simulink model "RobotX_ss_acousticsSingle_Dock_1023"  (R2014a)
settings: Solver=FixedStepDiscrete  StartTime=0.0  StopTime=inf  FixedStep=.25  RelTol=1e-3
undefined symbols (not defined in the file): Com1, Com2, Com3, Com4, DiscIntNeverNeededParam, standard
libraries: xpcseriallib x42, slrtlib x7, simulink x6, speedgoatlib x2, dspmtrx3 x1, speedgoatlib_IO102 x1
(part 4 of 4)

== matlab function RobotX_ss_acousticsSingle_Dock_1023/Sensors/1021 Comms/Message Selector/HRTSEA Message/MATLAB Function ==
  data: Time input; HRTLat input; HRTLong input; HRTTask input; HRTMode input; SEAValid input; asciiHRTSEA output; SEALat input; SEALong input; SEAColor input; SEADepth input
function asciiHRTSEA = asciiHRTSEAEncoder(Time,HRTLat,HRTLong,HRTTask,HRTMode,SEAValid,SEALat,SEALong,SEAColor,SEADepth)

% Initialize output message vector as the serial output block expects 128
% character message
asciiHRTSEA = uint8(zeros(1,128));

asciiComma = uint8(',');
asciiDeciPt = uint8('.');
asciiTeamID = uint8('FAUVU,');
asciiMsgEnd = uint8('*');
asciiMsgCRLF = [13 10];

% Convert UTC Time input (hhmmss) into ascii code
asciiTime = uint8(zeros(1,7));
asciiTime(7) = asciiComma;

for timeChar = 1:6
    asciiTime(timeChar) = floor(mod(Time,10^(7-timeChar))/...
        10^(6-timeChar)) + 48;
end

%%%%%%%%%%%%%%%%%%%%%%%%%%%%%%%%%%%%%%%%%%%%%%%%%%%%%%%%%%%%%%%%%%%%
% Heartbeat message
% Convert static strings to ascii code
asciiHRTMsgID = uint8('$RXHRT,');
if HRTLat >= 0
    asciiHRTNS = uint8('N,');
else
    HRTLat = -HRTLat;
    asciiHRTNS = uint8('S,');
end
if HRTLong >= 0
    asciiHRTEW = uint8('E,');
else
    HRTLong = -HRTLong;
    asciiHRTEW = uint8('W,');
end

% Convert latitude (dd.mmmmmm) into ascii code
asciiHRTLat = uint8(zeros(1,10));
asciiHRTLat(10) = asciiComma;
asciiHRTLat(3) = asciiDeciPt;

HRTlatInt = floor(HRTLat);
for latIntChar = 1:2
    asciiHRTLat(latIntChar) = floor(mod(HRTlatInt,10^(3-latIntChar))/...
        10^(2-latIntChar)) + 48;
end

HRTlatDeci = mod(HRTLat,HRTlatInt) * 10^6;
for latDeciChar = 1:6
    asciiHRTLat(latDeciChar+3) = floor(mod(HRTlatDeci,10^(7-latDeciChar))/...
        10^(6-latDeciChar)) + 48;
end

% Convert longitude (ddd.mmmmmm) into ascii code
asciiHRTLong = uint8(zeros(1,11));
asciiHRTLong(11) = asciiComma;
asciiHRTLong(4) = asciiDeciPt;

HRTlongInt = floor(HRTLong);
for longIntChar = 1:3
    asciiHRTLong(longIntChar) = floor(mod(HRTlongInt,10^(4-longIntChar))/...
        10^(3-longIntChar)) + 48;
end

HRTlongDeci = mod(HRTLong,HRTlongInt) * 10^6;
for longDeciChar = 1:6
    asciiHRTLong(longDeciChar+4) = floor(mod(HRTlongDeci,10^(7-longDeciChar))/...
        10^(6-longDeciChar)) + 48;
end

% Convert vehicle mode into ascii (1 = RC, 2 = Auto)

% Auto On 
if HRTMode == 3 
    HRTOpMode = 2;
    asciiHRTMode = [uint8(HRTOpMode+48) asciiComma];
else
    HRTOpMode = 1;
    asciiHRTMode = [uint8(HRTOpMode+48) asciiComma];
end

% Convert vehicle task into ascii
HRTTask = HRTTask - 1; % FSM: Init = 1, SSGate = 2, SEA = 3, Dock = 4, LIT = 5, Obst = 6
if HRTTask ~= 1 || 2 || 3 || 4 || 5
    HRTOpTask = 1;
    asciiHRTTask = [uint8(HRTOpTask+48) asciiMsgEnd];
else
    asciiHRTTask = [uint8(HRTTask+48) asciiMsgEnd];
end

% Concat individual ascii arrays into one array
asciiHRTPreChkSum = cat(2,asciiHRTMsgID,asciiTime,asciiHRTLat,asciiHRTNS,asciiHRTLong,asciiHRTEW,...
    asciiTeamID,asciiHRTMode,asciiHRTTask);

% Calculate the checksum of the message from the '$' to the '*' and convert
% to hex
HRTchkSum = uint8(0);

for chksumChar = 1:(length(asciiHRTPreChkSum)-2)
    HRTchkSum = bitxor(HRTchkSum,asciiHRTPreChkSum(chksumChar+1));
end

% Convert the checksum to ascii
HRTchkSum = dec2hex(HRTchkSum);
asciiHRTChkSum = uint8(zeros(1,length(HRTchkSum))+32);
for i = 1:length(HRTchkSum)
    asciiHRTChkSum(i) = uint8(HRTchkSum(i));
end

% Concat the checksum and the '/r/n' to the end of the message
asciiHRTPostChkSum = cat(2,asciiHRTPreChkSum,asciiHRTChkSum,asciiMsgCRLF);

%%%%%%%%%%%%%%%%%%%%%%%%%%%%%%%%%%%%%%%%%%%%%%%%%%%%%%%%%%%%%%%%%%%%%

% Underwater search message
asciiSEAMsgID = uint8('$RXSEA,');
if SEAValid == 1
    if SEALat >= 0
        asciiSEANS = uint8('N,');
    else
        SEALat = -SEALat;
        asciiSEANS = uint8('S,');
    end
    if SEALong >= 0
        asciiSEAEW = uint8('E,');
    else
        SEALong = -SEALong;
        asciiSEAEW = uint8('W,');
    end
else
    asciiSEANS = [32 asciiComma];
    asciiSEAEW = [32 asciiComma];
end

% Convert buoy color to ascii code (1 = R, 2 = G, 3 = B, 4 = W, 5 = K)
asciiSEAColor = [uint8(32) asciiComma]; % Initialize as whitespace in case no buoy is found

if SEAColor == 1
    asciiSEAColor(1) = uint8('R');
elseif SEAColor == 2
    asciiSEAColor(1) = uint8('G');
elseif SEAColor == 3
    asciiSEAColor(1) = uint8('B');
elseif SEAColor == 4
    asciiSEAColor(1) = uint8('W');
elseif SEAColor == 5
    asciiSEAColor(1) = uint8('K');
end

% Convert latitude (dd.mmmmmm) into ascii code
asciiSEALat = uint8(zeros(1,10)+32); % Initialize as whitespace in case no buoy is found
asciiSEALat(10) = asciiComma;

% Only output values if valid bit is high
if SEAValid == 1
    asciiSEALat(3) = asciiDeciPt;
    SEAlatInt = floor(SEALat);
    for latIntChar = 1:2
        asciiSEALat(latIntChar) = floor(mod(SEAlatInt,10^(3-latIntChar))/...
            10^(2-latIntChar)) + 48;
    end
    
    SEAlatDeci = mod(SEALat,SEAlatInt) * 10^6;
    for latDeciChar = 1:6
        asciiSEALat(latDeciChar+3) = floor(mod(SEAlatDeci,10^(7-latDeciChar))/...
            10^(6-latDeciChar)) + 48;
    end
end

% Convert longitude (ddd.mmmmmm) into ascii code
asciiSEALong = uint8(zeros(1,11)+32); % Initialize as whitespace in case no buoy is found
asciiSEALong(11) = asciiComma;

% Only output values if valid bit is high
if SEAValid == 1
    asciiSEALong(4) = asciiDeciPt;
    SEAlongInt = floor(SEALong);
    for longIntChar = 1:3
        asciiSEALong(longIntChar) = floor(mod(SEAlongInt,10^(4-longIntChar))/...
            10^(3-longIntChar)) + 48;
    end
    
    SEAlongDeci = mod(SEALong,SEAlongInt) * 10^6;
    for longDeciChar = 1:6
        asciiSEALong(longDeciChar+4) = floor(mod(SEAlongDeci,10^(7-longDeciChar))/...
            10^(6-longDeciChar)) + 48;
    end
end

% Convert depth (m) (##.##) into ascii
asciiSEADepth = uint8(zeros(1,6)+32); % Initialize as whitespace in case no buoy is found
asciiSEADepth(6) = asciiMsgEnd;

% Only output values if valid bit is high
if SEAValid == 1
    asciiSEADepth(3) = asciiDeciPt;
    SEAdepthInt = floor(SEADepth);
    for depthIntChar = 1:2
        asciiSEADepth(depthIntChar) = floor(mod(SEAdepthInt,10^(3-depthIntChar))/...
            10^(2-depthIntChar)) + 48;
    end
    
    SEAdepthDeci = mod(SEADepth,SEAdepthInt) * 10^2;
    for depthDeciChar = 1:2
        asciiSEADepth(depthDeciChar+3) = floor(mod(SEAdepthDeci,10^(3-depthDeciChar))/...
            10^(2-depthDeciChar)) + 48;
    end
end

% Concat individual ascii arrays into one array
asciiSEAPreChkSum = cat(2,asciiSEAMsgID,asciiTime,asciiTeamID,asciiSEAColor,...
    asciiSEALat,asciiSEANS,asciiSEALong,asciiSEAEW,asciiSEADepth);

% Calculate the checksum of the message from the '$' to the '*' and convert
% to hex
SEAchkSum = uint8(0);

for chksumChar = 1:(length(asciiSEAPreChkSum)-2)
    SEAchkSum = bitxor(SEAchkSum,asciiSEAPreChkSum(chksumChar+1));
end

% Convert the checksum to ascii
SEAchkSum = dec2hex(SEAchkSum);
asciiSEAChkSum = uint8(zeros(1,length(SEAchkSum))+32);
for i = 1:length(SEAchkSum)
    asciiSEAChkSum(i) = uint8(SEAchkSum(i));
end

% Concat the checksum and the '/r/n' to the end of the message
asciiSEAPostChkSum = cat(2,asciiSEAPreChkSum,asciiSEAChkSum,asciiMsgCRLF);

%%%%%%%%%%%%%%%%%%%%%%%%%%%%%%%%%%%%%%%%%%%%%%%%%%%%%%%%%%%%%%%%%%%%%%

asciiHRTSEAPostChkSum = cat(2,asciiHRTPostChkSum,asciiSEAPostChkSum);
asciiHRTSEA(1:length(asciiHRTSEAPostChkSum)) = asciiHRTSEAPostChkSum;

== matlab function RobotX_ss_acousticsSingle_Dock_1023/Sensors/1021 Comms/Pi Nav Send/Data Update1 ==
  data: Valid input; ControlMode input; V output; C output; L output; A output; Data input; D1 output; D2 output; D3 output; D4 output; D5 output; D6 output; D7 output; D8 output; D9 output; D10 output; D11 output; D12 output; D13 output; D14 output; D15 output; D16 output; D17 output; D18 output; D19 output; D20 output; D21 output; D22 output; D23 output; D24 output; Activate input
function [V,C,L,A,D1,D2,D3,D4,D5,D6,D7,D8,D9,D10,D11,D12,D13,D14,D15,D16,D17,...
    D18,D19,D20,D21,D22,D23,D24] = dataSplit(Valid,ControlMode,Data,Activate)
%Written by Anderson Lebbad on August 10, 2014
%Last Edited by: Anderson Lebbad on September 11, 2014

%This function splits the data vector into the twelve channels it is
%composed of for communication

persistent HoldData

A = Activate;

if isempty(HoldData)
    HoldData = zeros(26,1);
end

L = 8;

if Valid == 1
    HoldData(1) = Valid;
    HoldData(2) = ControlMode;
    HoldData(3) = Data(1);
    HoldData(4) = Data(2);
    HoldData(5) = Data(3);
    HoldData(6) = Data(4);
    HoldData(7) = Data(5);
    HoldData(8) = Data(6);
    HoldData(9) = Data(7);
    HoldData(10) = Data(8);
    HoldData(11) = Data(9);
    HoldData(12) = Data(10);
    HoldData(13) = Data(11);
    HoldData(14) = Data(12);
    HoldData(15) = Data(13);
    HoldData(16) = Data(14);
    HoldData(17) = Data(15);
    HoldData(18) = Data(16);
    HoldData(19) = Data(17);
    HoldData(20) = Data(18);
    HoldData(21) = Data(19);
    HoldData(22) = Data(20);
    HoldData(23) = Data(21);
    HoldData(24) = Data(22);
    HoldData(25) = Data(23);
    HoldData(26) = Data(24);
end

V = HoldData(1);
C = HoldData(2);
D1 = HoldData(3);
D2 = HoldData(4);
D3 = HoldData(5);
D4 = HoldData(6);
D5 = HoldData(7);
D6 = HoldData(8);
D7 = HoldData(9);
D8 = HoldData(10);
D9 = HoldData(11);
D10 = HoldData(12);
D11 = HoldData(13);
D12 = HoldData(14);
D13 = HoldData(15);
D14 = HoldData(16);
D15 = HoldData(17);
D16 = HoldData(18);
D17 = HoldData(19);
D18 = HoldData(20);
D19 = HoldData(21);
D20 = HoldData(22);
D21 = HoldData(23);
D22 = HoldData(24);
D23 = HoldData(25);
D24 = HoldData(26);

end

== matlab function RobotX_ss_acousticsSingle_Dock_1023/Main FSM/Acoustic Single Point FSM/Main Enabler ==
  data: taskSelector output; MoveEn output; Acoustic1En output; ReportEn output; MoveFin input; AcousticFin input
function [taskSelector,MoveEn,Acoustic1En,ReportEn] = taskEnabler(MoveFin,AcousticFin)
%Written by Anderson Lebbad on July 19, 2013
%Last Edited: Anderson Lebbad on October 22, 2014
%
%   Substring search for task was written in
%   Case switches were redundant, combined with first set of if statements
%
%   Most recent edit simplifies to single point orientation.

%Changes the value of MainMode and the enablers for the tasks within the
%Main FSM.

% Initialize enable signals
MoveEn = 0;
Acoustic1En = 0;
ReportEn = 0;

% Set enable signals based on state completion
if MoveFin == 0
    MoveEn = 1;
    taskSelector = 1;
elseif AcousticFin == 0
    Acoustic1En = 1;
    taskSelector = 2;
else
    ReportEn = 1;
    taskSelector = 7;
end

== matlab function RobotX_ss_acousticsSingle_Dock_1023/Main FSM/Acoustic Single Point FSM/Move/CalcTimes ==
  data: pts input; u input; Data output
function Data = calcTimes(pts, u)
%Written by Anderson Lebbad on August 9, 2014
%Last Edited: Dylan DeGaetano September 1, 2014

%Calculates times for the boat to get to points for a trajectory, and
%formats Data for communication

%Initialize
Data = zeros(24,1);
traj = zeros(8,3);
traj(:,1:2) = pts;



for k = 2:8
    %Calculate distance to travel from last point
    distTravel = sqrt(sum((pts(k-1,:)-pts(k,:)).^2));
    %Assume 1m per second speed
    traj(k,3) = traj(k-1,3) + distTravel;
    %Add time based off initial velocity to get to first point past initial
    if k == 2
        traj(k,3) = traj(k,3) + 2.5*abs(2-u);
    end
end


%Output Data
for i=1:8
    for j = 1:3
        Data(3*(i-1)+j) = traj(i,j);
    end
end

== matlab function RobotX_ss_acousticsSingle_Dock_1023/Main FSM/Acoustic Single Point FSM/Move/GPSMove ==
  data: GoalNED input; X input; Finished output; valid output; Y input; Psi input; pts output
function [Finished,valid,pts] = GPSmove(GoalNED,X,Y,Psi)
%Written by Dylan DeGaetano on September 1, 2014
%Last edited by: Anderson Lebbad
%
%This function will go to a given NED cooridnate, last edit changed the
%goal pt and variable names

persistent Sample
if isempty(Sample)
Sample = 0;
end
Finished = 0;
pts = zeros(8,2);
%$Distance to object in meters
if Sample >= 100
    Sample = 0;
end

if Sample == 0
    pts(1,1) = X+5*cos(Psi*pi/180);
    pts(1,2) = Y+5*sin(Psi*pi/180);
    pts(8,1) = GoalNED(1,1);
    pts(8,2) = GoalNED(1,2);
    pts(2,:) = pts(1,:) +(1*(GoalNED-pts(1,:))/7);
    pts(3,:) = pts(1,:) +(2*(GoalNED-pts(1,:))/7);
    pts(4,:) = pts(1,:) +(3*(GoalNED-pts(1,:))/7);
    pts(5,:) = pts(1,:) +(4*(GoalNED-pts(1,:))/7);
    pts(6,:) = pts(1,:) +(5*(GoalNED-pts(1,:))/7);
    pts(7,:) = pts(1,:) +(6*(GoalNED-pts(1,:))/7);
    Sample = 1; 
    valid = 1;
    
else 
    range = sqrt(sum((GoalNED - [X Y]).^2));
    if range <= 5
        Finished = 1;
    end
    valid = 0;
    Sample = Sample + 1;
end

== matlab function RobotX_ss_acousticsSingle_Dock_1023/Course Selections/MATLAB Function ==
  data: Course input; StartGPS output; AStartGPS input; AssGateGPS input; AacouGPS input; AdockGPS input; AltGPS input; AodoaGPS input; Afreq input; Arate input; Aoffset input; Asymbol input; AODOAentry input; AODOAexit input; AfinishGPS input; BStartGPS input; BssGateGPS input; BacouGPS input; BdockGPS input; BltGPS input; BodoaGPS input; Bfreq input; Brate input; Boffset input; Bsymbol input; BODOAentry input; BODOAexit input; BfinishGPS input; TStartGPS input; TssGateGPS input; TacouGPS input; TdockGPS input; TltGPS input; TodoaGPS input; Tfreq input; Trate input; Toffset input; Tsymbol input; TODOAentry input; TODOAexit input; ssGateGPS output; acouGPS output; dockGPS output; ltGPS output; odoaGPS output; freq output; rate output; offset output; symbol output; ODOAentry output; ODOAexit output; TfinishGPS input; finishGPS output
function [StartGPS,ssGateGPS,acouGPS,dockGPS,ltGPS,odoaGPS,freq,rate,offset,symbol,ODOAentry,ODOAexit,finishGPS]...
    = fcn(Course,AStartGPS,AssGateGPS,AacouGPS,AdockGPS,AltGPS,AodoaGPS,Afreq,Arate,Aoffset,Asymbol,AODOAentry,AODOAexit,AfinishGPS,...
    BStartGPS,BssGateGPS,BacouGPS,BdockGPS,BltGPS,BodoaGPS,Bfreq,Brate,Boffset,Bsymbol,BODOAentry,BODOAexit,BfinishGPS,...
    TStartGPS,TssGateGPS,TacouGPS,TdockGPS,TltGPS,TodoaGPS,Tfreq,Trate,Toffset,Tsymbol,TODOAentry,TODOAexit,TfinishGPS)

%Written by Anderson Lebbbad on October 19, 2014
%Last Edited by:
%
%This function switches between stored GPS points based upon the selected
%course letter.

switch(Course)
    case uint8('A')
        StartGPS = AStartGPS;
        ssGateGPS = AssGateGPS;
        acouGPS = AacouGPS;
        dockGPS = AdockGPS;
        ltGPS = AltGPS;
        odoaGPS = AodoaGPS;
        freq = Afreq;
        rate = Arate;
        offset = Aoffset;
        symbol = Asymbol;
        ODOAentry = AODOAentry;
        ODOAexit = AODOAexit;
        finishGPS = AfinishGPS;
    case uint8('B')
        StartGPS = BStartGPS;
        ssGateGPS = BssGateGPS;
        acouGPS = BacouGPS;
        dockGPS = BdockGPS;
        ltGPS = BltGPS;
        odoaGPS = BodoaGPS;
        freq = Bfreq;
        rate = Brate;
        offset = Boffset;
        symbol = Bsymbol;
        ODOAentry = BODOAentry;
        ODOAexit = BODOAexit;
        finishGPS = BfinishGPS;
    otherwise
        StartGPS = TStartGPS;
        ssGateGPS = TssGateGPS;
        acouGPS = TacouGPS;
        dockGPS = TdockGPS;
        ltGPS = TltGPS;
        odoaGPS = TodoaGPS;
        freq = Tfreq;
        rate = Trate;
        offset = Toffset;
        symbol = Tsymbol;
        ODOAentry = TODOAentry;
        ODOAexit = TODOAexit;
        finishGPS = TfinishGPS;
end

end

== matlab function RobotX_ss_acousticsSingle_Dock_1023/Sensors/1021 Comms/Message Selector/MATLAB Function ==
  data: taskNumber input; messageNumber output
function messageNumber = messageSelector(taskNumber)

% FSM Task Number 
%   1 = Initialization 
%   2 = ss gate 
%   3 = Acoustic Detection
%   4 = Docking 
%   5 = Light Tower Detection 
%   6 = Obstacle Field 

% Comms Task Number 
% 2 = Acoustic Detection
% 3 = Light tower

% Acoustic Task 
if taskNumber-1 == 2
    messageNumber = 2;
% Light Tower Task 
elseif taskNumber-1 == 4
    messageNumber = 3;
% Default Heart Beat 
else
    messageNumber = 1;
end

== matlab function RobotX_ss_acousticsSingle_Dock_1023/Main FSM/Start//Speedgate/GPS Move/CalcTimes ==
  data: pts input; u input; Data output
function Data = calcTimes(pts, u)
%Written by Anderson Lebbad on August 9, 2014
%Last Edited: Dylan DeGaetano September 1, 2014

%Calculates times for the boat to get to points for a trajectory, and
%formats Data for communication

%Initialize
Data = zeros(24,1);
traj = zeros(8,3);
traj(:,1:2) = pts;



for k = 2:8
    %Calculate distance to travel from last point
    distTravel = sqrt(sum((pts(k-1,:)-pts(k,:)).^2));
    %Assume 1m per second speed
    traj(k,3) = traj(k-1,3) + distTravel;
    %Add time based off initial velocity to get to first point past initial
    if k == 2
        traj(k,3) = traj(k,3) + 2.5*abs(2-u);
    end
end


%Output Data
for i=1:8
    for j = 1:3
        Data(3*(i-1)+j) = traj(i,j);
    end
end

== matlab function RobotX_ss_acousticsSingle_Dock_1023/Main FSM/Start//Speedgate/GPS Move/GPSMove ==
  data: GoalNED input; X input; Finished output; valid output; Y input; Psi input; pts output
function [Finished,valid,pts] = GPSmove(GoalNED,X,Y,Psi)
%Written by Dylan DeGaetano on September 1, 2014
%Last edited by: Anderson Lebbad
%
%This function will go to a given NED cooridnate, last edit changed the
%goal pt and variable names

persistent Sample
if isempty(Sample)
Sample = 0;
end
Finished = 0;
pts = zeros(8,2);
%$Distance to object in meters
if Sample >= 100
    Sample = 0;
end

if Sample == 0
    pts(1,1) = X+5*cos(Psi*pi/180);
    pts(1,2) = Y+5*sin(Psi*pi/180);
    pts(8,1) = GoalNED(1,1);
    pts(8,2) = GoalNED(1,2);
    pts(2,:) = pts(1,:) +(1*(GoalNED-pts(1,:))/7);
    pts(3,:) = pts(1,:) +(2*(GoalNED-pts(1,:))/7);
    pts(4,:) = pts(1,:) +(3*(GoalNED-pts(1,:))/7);
    pts(5,:) = pts(1,:) +(4*(GoalNED-pts(1,:))/7);
    pts(6,:) = pts(1,:) +(5*(GoalNED-pts(1,:))/7);
    pts(7,:) = pts(1,:) +(6*(GoalNED-pts(1,:))/7);
    Sample = 1; 
    valid = 1;
    
else 
    range = sqrt(sum((GoalNED - [X Y]).^2));
    if range <= 8
        Finished = 1;
    end
    valid = 0;
    Sample = Sample + 1;
end

== matlab function RobotX_ss_acousticsSingle_Dock_1023/Main FSM/Start//Speedgate/GPS Move/LLA to NED ==
  data: LLA input; GoalNED output; NED_origin input
function GoalNED = LLA2NEDfun(LLA,NED_origin)
%Written by Anderson Lebbad on September 20, 2014
%Last edited by:
%
%This function converts a target Latitude, Longitude, Altitude (LLA) point
%into North, East, Down (NED) coordinates

%First convert to earth centered, earth fixed frame
GoalECEF = lla2ecef([LLA*(pi/180), 0]');
%Then convert from ECEF to North East Down
GoalNEDvect = ecef2ned(NED_origin'*(pi/180),GoalECEF);
GoalNED = GoalNEDvect(1:2)';


end

function x_ecef = lla2ecef(x_lla)
% LLE2ECEF: Converts from geodetic latitude, longitude, and altitude to earth-centered earth-fixed Cartesian coordinates
% INPUT: latitude phi (rad), longitude lambda (rad), altitude h (m)
% OUTPUT: [x, y, z]' (m) earth-centered earth-fixed Cartesian coordinates
    a = 6378137; % equatorial radius of ellipsoid (semi-major axis) (m)
    b = 6356752; % polar axis radius of ellipsoid (semi-minor axis) (m)

    phi = x_lla(1);
    lambda = x_lla(2);
    h = x_lla(3);
    
    % auxiliar quantities f, e, and N
    f = (a-b)/a;
    e = f*(2-f);
    N = a/sqrt(1-(e*sin(phi))^2);
    x_ecef = [(N+h)*cos(phi)*cos(lambda); (N+h)*cos(phi)*sin(lambda); (N*(1-e^2)+h)*sin(phi)];
end

function [x_ned] = ecef2ned(ned_lla, x_ecef)
% ECEF2NED Converts from earth-centered, earth-fixed Cartesian coordinates to tangent plane
% INPUT:
% 1) x_ecef=[x,y,z]' (m) earth-centered, earth-fixed Cartesian coordinates
% 2) ned_lla=[phi,lambda]' consiting of latitude phi (rad), longitude lambda (rad) of NED origin
% OUTPUT:
% 1) x_ned=[x,y,z]' (m) in NED coordinate system with the origin [phi,lambda]'

    phi = ned_lla(1);
    lambda = ned_lla(2);

    % transformation  matrix
    T = [-sin(phi)*cos(lambda) -sin(phi)*sin(lambda)  cos(phi)
         -sin(lambda)           cos(lambda)           0
          cos(phi)*cos(lambda)   cos(phi)*sin(lambda)  sin(phi)];

     x_ned = T*(x_ecef-lla2ecef([phi, lambda, 0]')); % convert to NED
     x_ned(3) = -x_ned(3);
end

== matlab function RobotX_ss_acousticsSingle_Dock_1023/Main FSM/Start//Speedgate/Main Enabler ==
  data: taskSelector output; GpsEn output; entEn output; exitEn output; ssgateTask input; GpsFin input; entFin input
function [taskSelector,GpsEn,entEn,exitEn]=Startgate_Enabler(ssgateTask,...
    GpsFin,entFin)
%Written by Anderson Lebbad on July 19, 2013
%Last Edited: Dylan DeGaetano on September ,4 2014
%   Substring search for task was written in
%   Case switches were redundant, combined with first set of if statements

%Changes the value of MainMode and the enablers for the tasks within the
%Main FSM.

% Initialize enable signals
GpsEn = 0;
entEn =0;
exitEn = 0;

% Convert main task indicator to a string
ssgateTaskStr = char(ssgateTask);

% Adjust finished states based on user task selection (never skips
% initialization)
if ~isempty(strfind(ssgateTaskStr,'Aim'))
    GpsFin = 1;
elseif ~isempty(strfind(ssgateTaskStr,'Start'))
    GpsFin = 1;
    entFin = 1;
elseif ~isempty(strfind(ssgateTaskStr,'Speed'))
    GpsFin = 1;
    entFin = 1;
end

% Set enable signals based on state completion
if GpsFin == 0
    GpsEn = 1;
    taskSelector = 1;
elseif entFin == 0
    entEn = 1;
    taskSelector = 2;
else
    exitEn = 1;
    taskSelector = 3;
end

== matlab function RobotX_ss_acousticsSingle_Dock_1023/Main FSM/Termination/CalcTimes ==
  data: pts input; u input; Data output
function Data = calcTimes(pts, u)
%Written by Anderson Lebbad on August 9, 2014
%Last Edited: Dylan DeGaetano September 1, 2014

%Calculates times for the boat to get to points for a trajectory, and
%formats Data for communication

%Initialize
Data = zeros(24,1);
traj = zeros(8,3);
traj(:,1:2) = pts;



for k = 2:8
    %Calculate distance to travel from last point
    distTravel = sqrt(sum((pts(k-1,:)-pts(k,:)).^2));
    %Assume 1m per second speed
    traj(k,3) = traj(k-1,3) + distTravel;
    %Add time based off initial velocity to get to first point past initial
    if k == 2
        traj(k,3) = traj(k,3) + 2.5*abs(2-u);
    end
end


%Output Data
for i=1:8
    for j = 1:3
        Data(3*(i-1)+j) = traj(i,j);
    end
end

== matlab function RobotX_ss_acousticsSingle_Dock_1023/Sensors/1021 Comms/Message Selector/HRTSEA Message/MATLAB Function1 ==
  data: pingerInfo input; SEAValid output; SEALat output; SEALong output; SEAColor output; SEADepth output
function [SEAValid,SEALat,SEALong,SEAColor,SEADepth] = pingerInfoParse(pingerInfo)

SEAValid = pingerInfo(1);
SEALat = pingerInfo(2);
SEALong = pingerInfo(3);
SEADepth = pingerInfo(4);
SEAColor = pingerInfo(5);

== matlab function RobotX_ss_acousticsSingle_Dock_1023/Sensors/1021 Comms/Message Selector/HRTLIT Message/MATLAB Function1 ==
  data: ltSeq input; LITValid output; LITSequence output
function [LITValid,LITSequence] = LITSeqParse(ltSeq)

LITValid = ltSeq(1);
LITSequence = ltSeq(2:4);

== matlab function RobotX_ss_acousticsSingle_Dock_1023/Sensors/1021 Comms/Pi Nav Send/Data Update2 ==
  data: Valid input; ControlMode input; V output; C output; L output; A output; Data input; D1 output; D2 output; D3 output; D4 output; D5 output; D6 output; D7 output; D8 output; D9 output; D10 output; D11 output; D12 output; D13 output; D14 output; D15 output; D16 output; D17 output; D18 output; D19 output; D20 output; D21 output; D22 output; D23 output; D24 output; Activate input
function [V,C,L,A,D1,D2,D3,D4,D5,D6,D7,D8,D9,D10,D11,D12,D13,D14,D15,D16,D17,...
    D18,D19,D20,D21,D22,D23,D24] = dataSplit(Valid,ControlMode,Data,Activate)
%Written by Anderson Lebbad on August 10, 2014
%Last Edited by: Anderson Lebbad on September 11, 2014

%This function splits the data vector into the twelve channels it is
%composed of for communication

persistent HoldData

if isempty(HoldData)
    HoldData = zeros(26,1);
    HoldData(2) = 2;
end

if Valid == 1
    HoldData(1) = Valid;
    HoldData(2) = ControlMode;
    HoldData(3) = Data(1);
    HoldData(4) = Data(2);
    HoldData(5) = Data(3);
    HoldData(6) = Data(4);
    HoldData(7) = Data(5);
    HoldData(8) = Data(6);
    HoldData(9) = Data(7);
    HoldData(10) = Data(8);
    HoldData(11) = Data(9);
    HoldData(12) = Data(10);
    HoldData(13) = Data(11);
    HoldData(14) = Data(12);
    HoldData(15) = Data(13);
    HoldData(16) = Data(14);
    HoldData(17) = Data(15);
    HoldData(18) = Data(16);
    HoldData(19) = Data(17);
    HoldData(20) = Data(18);
    HoldData(21) = Data(19);
    HoldData(22) = Data(20);
    HoldData(23) = Data(21);
    HoldData(24) = Data(22);
    HoldData(25) = Data(23);
    HoldData(26) = Data(24);
end

V = HoldData(1);
C = HoldData(2);
L = 8;
A = Activate;
D1 = HoldData(3);
D2 = HoldData(4);
D3 = HoldData(5);
D4 = HoldData(6);
D5 = HoldData(7);
D6 = HoldData(8);
D7 = HoldData(9);
D8 = HoldData(10);
D9 = HoldData(11);
D10 = HoldData(12);
D11 = HoldData(13);
D12 = HoldData(14);
D13 = HoldData(15);
D14 = HoldData(16);
D15 = HoldData(17);
D16 = HoldData(18);
D17 = HoldData(19);
D18 = HoldData(20);
D19 = HoldData(21);
D20 = HoldData(22);
D21 = HoldData(23);
D22 = HoldData(24);
D23 = HoldData(25);
D24 = HoldData(26);

end

== matlab function RobotX_ss_acousticsSingle_Dock_1023/Sensors/1021 Comms/UTC Timer/MATLAB Function ==
  data: inTime input; timeOut output
function timeOut  = UTCtimer(inTime)
% This script works as a timer in UTC time (hhmmss) for the boat

persistent startTime

if isempty(startTime)
    startTime = inTime;
end

    hours = floor(startTime/10000);
    minutes = floor(mod(startTime,10000)/100);
    seconds = mod(startTime,100);
    
    if seconds > 59
        minutes = minutes + 1;
        seconds = 0;
    end
    
    if minutes > 59
        hours = hours + 1;
        minutes = 0;
    end
    
    if hours > 23
        hours = 0;
    end
    
    startTime = hours * 10000 + minutes * 100 + seconds;
    
    timeOut = floor(startTime);
    
    startTime = startTime + 0.25;

== matlab function RobotX_ss_acousticsSingle_Dock_1023/Main FSM/Docking/Dock Enabler ==
  data: taskSelector output; GpsEn output; DockEn output; ReverseEn output; mainTask input; GpsFin input; DockFin input
function [taskSelector,GpsEn,DockEn,ReverseEn]=Dock_Enabler(mainTask,GpsFin,DockFin)
%Written by Anderson Lebbad on July 19, 2013
%Last Edited: Dylan DeGaetano on September ,4 2014
%   Substring search for task was written in
%   Case switches were redundant, combined with first set of if statements

%Changes the value of MainMode and the enablers for the tasks within the
%Main FSM.

% Initialize enable signals
GpsEn = 0;
DockEn = 0;
ReverseEn = 0; % Enable reverse out of docking bay 

% Convert main task indicator to a string
mainTaskStr = char(mainTask);

% Adjust finished states based on user task selection (never skips
% initialization)
if ~isempty(strfind(mainTaskStr,'Dock'))
    GpsFin = 1;
elseif ~isempty(strfind(mainTaskStr,'reverse'))
    GpsFin = 1;
    DockFin = 1;
end

% Set enable signals based on state completion
% Not at GPS Initial Point Yet, so get to Pt first
if GpsFin == 0
    GpsEn = 1;
    taskSelector = 1;
% Not Docked yet, so do Dock Enable  
elseif DockFin == 0
    DockEn = 1;
    taskSelector = 2;
% Reverse Wam-v from dock
else
    ReverseEn = 1 ;
    taskSelector = 3;
end

== matlab function RobotX_ss_acousticsSingle_Dock_1023/Main FSM/Docking/Docking/LLA to NED ==
  data: Course input; LLAs input; GoalNED output; NED_origin input
function GoalNED = LLA2NEDfun(Course,LLAs,NED_origin)
%Written by Anderson Lebbad on September 20, 2014
%Last edited by:
%
%This function converts a target Latitude, Longitude, Altitude (LLA) point
%into North, East, Down (NED) coordinates

NED  = zeros(4,2);
for i=1:4
%First convert to earth centered, earth fixed frame
GoalECEF = lla2ecef([LLAs(i,:)*(pi/180), 0]');
%Then convert from ECEF to North East Down
GoalNEDvect = ecef2ned(NED_origin'*(pi/180),GoalECEF);
NED(i,:) = GoalNEDvect(1:2)';
end

GoalNED = sum(NED)/4;

if Course == uint8('T')
    GoalNED = LLAs(1,:);
end

end

function x_ecef = lla2ecef(x_lla)
% LLE2ECEF: Converts from geodetic latitude, longitude, and altitude to earth-centered earth-fixed Cartesian coordinates
% INPUT: latitude phi (rad), longitude lambda (rad), altitude h (m)
% OUTPUT: [x, y, z]' (m) earth-centered earth-fixed Cartesian coordinates
    a = 6378137; % equatorial radius of ellipsoid (semi-major axis) (m)
    b = 6356752; % polar axis radius of ellipsoid (semi-minor axis) (m)

    phi = x_lla(1);
    lambda = x_lla(2);
    h = x_lla(3);
    
    % auxiliar quantities f, e, and N
    f = (a-b)/a;
    e = f*(2-f);
    N = a/sqrt(1-(e*sin(phi))^2);
    x_ecef = [(N+h)*cos(phi)*cos(lambda); (N+h)*cos(phi)*sin(lambda); (N*(1-e^2)+h)*sin(phi)];
end

function [x_ned] = ecef2ned(ned_lla, x_ecef)
% ECEF2NED Converts from earth-centered, earth-fixed Cartesian coordinates to tangent plane
% INPUT:
% 1) x_ecef=[x,y,z]' (m) earth-centered, earth-fixed Cartesian coordinates
% 2) ned_lla=[phi,lambda]' consiting of latitude phi (rad), longitude lambda (rad) of NED origin
% OUTPUT:
% 1) x_ned=[x,y,z]' (m) in NED coordinate system with the origin [phi,lambda]'

    phi = ned_lla(1);
    lambda = ned_lla(2);

    % transformation  matrix
    T = [-sin(phi)*cos(lambda) -sin(phi)*sin(lambda)  cos(phi)
         -sin(lambda)           cos(lambda)           0
          cos(phi)*cos(lambda)   cos(phi)*sin(lambda)  sin(phi)];

     x_ned = T*(x_ecef-lla2ecef([phi, lambda, 0]')); % convert to NED
     x_ned(3) = -x_ned(3);
end

== matlab function RobotX_ss_acousticsSingle_Dock_1023/Main FSM/Docking/GPS Move/GPSMove ==
  data: GoalNED input; X input; Finished output; valid output; Y input; Psi input; pts output
function [Finished,valid,pts] = GPSmove(GoalNED,X,Y,Psi)
%Written by Dylan DeGaetano on September 1, 2014
%Last edited by: Anderson Lebbad
%
%This function will go to a given NED cooridnate, last edit changed the
%goal pt and variable names

% Input of GoalNED is a 10x2 matrix of NED coords where the first row is
% the coord of the docking observation point

persistent Sample
if isempty(Sample)
Sample = 0;
end
Finished = 0;
pts = zeros(8,2);
%$Distance to object in meters
if Sample == 100
    Sample = 0;
end

if Sample == 0
    pts(1,1) = X+5*cos(Psi*pi/180);
    pts(1,2) = Y+5*sin(Psi*pi/180);
    pts(8,1) = GoalNED(1,1);
    pts(8,2) = GoalNED(1,2);
    pts(2,:) = pts(1,:) +(1*(GoalNED(1,:)-pts(1,:))/7);
    pts(3,:) = pts(1,:) +(2*(GoalNED(1,:)-pts(1,:))/7);
    pts(4,:) = pts(1,:) +(3*(GoalNED(1,:)-pts(1,:))/7);
    pts(5,:) = pts(1,:) +(4*(GoalNED(1,:)-pts(1,:))/7);
    pts(6,:) = pts(1,:) +(5*(GoalNED(1,:)-pts(1,:))/7);
    pts(7,:) = pts(1,:) +(6*(GoalNED(1,:)-pts(1,:))/7);
    Sample = 1; 
    valid = 1;
    
else 
    range = sqrt(sum((GoalNED(1,:) - [X Y]).^2));
    if range <= 5
        Finished = 1;
    end
    valid = 0;
    Sample = Sample + 1;
end

== matlab function RobotX_ss_acousticsSingle_Dock_1023/Sensors/1020 Comms/Data Update1 ==
  data: Valid input; ControlMode input; V output; C output; L output; A output; Data input; D1 output; D2 output; D3 output; D4 output; D5 output; D6 output; D7 output; D8 output; D9 output; D10 output; D11 output; D12 output; D13 output; D14 output; D15 output; D16 output; D17 output; D18 output; D19 output; D20 output; D21 output; D22 output; D23 output; D24 output; Activate input
function [V,C,L,A,D1,D2,D3,D4,D5,D6,D7,D8,D9,D10,D11,D12,D13,D14,D15,D16,D17,...
    D18,D19,D20,D21,D22,D23,D24] = dataSplit(Valid,ControlMode,Data,Activate)
%Written by Anderson Lebbad on August 10, 2014
%Last Edited by: Anderson Lebbad on September 11, 2014

%This function splits the data vector into the twelve channels it is
%composed of for communication

persistent HoldData

A = Activate;

if isempty(HoldData)
    HoldData = zeros(26,1);
end

L = 8;

if Valid == 1
    HoldData(1) = Valid;
    HoldData(2) = ControlMode;
    HoldData(3) = Data(1);
    HoldData(4) = Data(2);
    HoldData(5) = Data(3);
    HoldData(6) = Data(4);
    HoldData(7) = Data(5);
    HoldData(8) = Data(6);
    HoldData(9) = Data(7);
    HoldData(10) = Data(8);
    HoldData(11) = Data(9);
    HoldData(12) = Data(10);
    HoldData(13) = Data(11);
    HoldData(14) = Data(12);
    HoldData(15) = Data(13);
    HoldData(16) = Data(14);
    HoldData(17) = Data(15);
    HoldData(18) = Data(16);
    HoldData(19) = Data(17);
    HoldData(20) = Data(18);
    HoldData(21) = Data(19);
    HoldData(22) = Data(20);
    HoldData(23) = Data(21);
    HoldData(24) = Data(22);
    HoldData(25) = Data(23);
    HoldData(26) = Data(24);
end

V = HoldData(1);
C = HoldData(2);
D1 = HoldData(3);
D2 = HoldData(4);
D3 = HoldData(5);
D4 = HoldData(6);
D5 = HoldData(7);
D6 = HoldData(8);
D7 = HoldData(9);
D8 = HoldData(10);
D9 = HoldData(11);
D10 = HoldData(12);
D11 = HoldData(13);
D12 = HoldData(14);
D13 = HoldData(15);
D14 = HoldData(16);
D15 = HoldData(17);
D16 = HoldData(18);
D17 = HoldData(19);
D18 = HoldData(20);
D19 = HoldData(21);
D20 = HoldData(22);
D21 = HoldData(23);
D22 = HoldData(24);
D23 = HoldData(25);
D24 = HoldData(26);

end

== matlab function RobotX_ss_acousticsSingle_Dock_1023/Sensors/1020 Comms/MATLAB Function2 ==
  data: Time input; asciiLIT output; Sequence input
% This function creates the light tower message to be sent from 
% Speedgoat in ascii code
% Written by: Edward Zhu
% Date: 9/17/14

function asciiLIT = asciiLITEncoder(Time, Sequence)

% Initialize output message vector as the serial output block expects 128
% character message
asciiLIT = uint8(zeros(1,128));

% Convert static strings to ascii code
asciiMsgID = uint8('$RXLIT,');
asciiComma = uint8(',');
asciiTeamID = uint8('FAUVU,');
asciiMsgEnd = uint8('*');
asciiMsgCRLF = [13 10];

% Convert UTC Time input (hhmmss) into ascii code
asciiTime = uint8(zeros(1,7));
asciiTime(7) = asciiComma;

for timeChar = 1:6
    asciiTime(timeChar) = floor(mod(Time,10^(7-timeChar))/...
        10^(6-timeChar)) + 48;
end

% Convert the light sequece into ascii code (1 = R, 2 = B, 3 = G)
asciiSeq = uint8(zeros(1,4)+32);
asciiSeq(4) = asciiMsgEnd;

if Sequence(1) > 0 && Sequence(2) > 0 && Sequence(3) > 0
    for seqChar = 1:3
        if Sequence(seqChar) == 1
            Sequence(seqChar) = uint8('R');
        elseif Sequence(seqChar) == 2
            Sequence(seqChar) = uint8('B');
        elseif Sequence(seqChar) == 3
            Sequence(seqChar) = uint8('G');
        end
    end
    asciiSeq(1:3) = Sequence;
end

% Concat individual ascii arrays into one array
asciiPreChkSum = cat(2,asciiMsgID,asciiTime,asciiTeamID,asciiSeq);

% Calculate the checksum of the message from the '$' to the '*' and convert
% to hex
chkSum = uint8(0);

for chksumChar = 1:(length(asciiPreChkSum)-2)
    chkSum = bitxor(chkSum,asciiPreChkSum(chksumChar+1));
end

% Convert the checksum to ascii
chkSum = dec2hex(chkSum);
asciiChkSum = uint8(zeros(1,length(chkSum))+32);
for i = 1:length(chkSum)
    asciiChkSum(i) = uint8(chkSum(i));
end

% Concat the checksum and the '/r/n' to the end of the message
asciiPostChkSum = cat(2,asciiPreChkSum,asciiChkSum,asciiMsgCRLF);

% Output the final message
asciiLIT(1:length(asciiPostChkSum)) = asciiPostChkSum;

== matlab function RobotX_ss_acousticsSingle_Dock_1023/Main FSM/Termination/GPSMove ==
  data: GoalNED input; X input; valid output; Y input; Psi input; pts output
function [valid,pts] = GPSmove(GoalNED,X,Y,Psi)
%Written by Dylan DeGaetano on September 1, 2014
%Last edited by: Anderson Lebbad
%
%This function will go to a given NED cooridnate, last edit changed the
%goal pt and variable names

persistent Sample
if isempty(Sample)
Sample = 0;
end

pts = zeros(8,2);
%$Distance to object in meters

if Sample == 0
    pts(1,1) = X+5*cos(Psi*pi/180);
    pts(1,2) = Y+5*sin(Psi*pi/180);
    pts(8,1) = GoalNED(1,1);
    pts(8,2) = GoalNED(1,2);
    pts(2,:) = pts(1,:) +(1*(GoalNED-pts(1,:))/7);
    pts(3,:) = pts(1,:) +(2*(GoalNED-pts(1,:))/7);
    pts(4,:) = pts(1,:) +(3*(GoalNED-pts(1,:))/7);
    pts(5,:) = pts(1,:) +(4*(GoalNED-pts(1,:))/7);
    pts(6,:) = pts(1,:) +(5*(GoalNED-pts(1,:))/7);
    pts(7,:) = pts(1,:) +(6*(GoalNED-pts(1,:))/7);
    Sample = 1; 
    valid = 1;
    
else
    valid = 0;
end

== matlab function RobotX_ss_acousticsSingle_Dock_1023/Main FSM/Termination/LLA to NED ==
  data: Course input; GoalLLA input; GoalNED output; NED_origin input
function GoalNED = LLA2NEDfun(Course,GoalLLA,NED_origin)
%Written by Anderson Lebbad on September 20, 2014
%Last edited by:
%
%This function converts a target Latitude, Longitude, Altitude (LLA) point
%into North, East, Down (NED) coordinates

%First convert to earth centered, earth fixed frame
GoalECEF1 = lla2ecef([GoalLLA(1,:)*(pi/180), 0]');
%Then convert from ECEF to North East Down
GoalNEDvect1 = ecef2ned(NED_origin'*(pi/180),GoalECEF1);
GoalNED1 = GoalNEDvect1(1:2)';

%First convert to earth centered, earth fixed frame
GoalECEF2 = lla2ecef([GoalLLA(2,:)*(pi/180), 0]');
%Then convert from ECEF to North East Down
GoalNEDvect2 = ecef2ned(NED_origin'*(pi/180),GoalECEF2);
GoalNED2 = GoalNEDvect2(1:2)';

GoalNED = (GoalNED1 + GoalNED2) / 2;

if Course == uint8('T')
    GoalNED = GoalLLA(1,:);
end

end

function x_ecef = lla2ecef(x_lla)
% LLE2ECEF: Converts from geodetic latitude, longitude, and altitude to earth-centered earth-fixed Cartesian coordinates
% INPUT: latitude phi (rad), longitude lambda (rad), altitude h (m)
% OUTPUT: [x, y, z]' (m) earth-centered earth-fixed Cartesian coordinates
    a = 6378137; % equatorial radius of ellipsoid (semi-major axis) (m)
    b = 6356752; % polar axis radius of ellipsoid (semi-minor axis) (m)

    phi = x_lla(1);
    lambda = x_lla(2);
    h = x_lla(3);
    
    % auxiliar quantities f, e, and N
    f = (a-b)/a;
    e = f*(2-f);
    N = a/sqrt(1-(e*sin(phi))^2);
    x_ecef = [(N+h)*cos(phi)*cos(lambda); (N+h)*cos(phi)*sin(lambda); (N*(1-e^2)+h)*sin(phi)];
end

function [x_ned] = ecef2ned(ned_lla, x_ecef)
% ECEF2NED Converts from earth-centered, earth-fixed Cartesian coordinates to tangent plane
% INPUT:
% 1) x_ecef=[x,y,z]' (m) earth-centered, earth-fixed Cartesian coordinates
% 2) ned_lla=[phi,lambda]' consiting of latitude phi (rad), longitude lambda (rad) of NED origin
% OUTPUT:
% 1) x_ned=[x,y,z]' (m) in NED coordinate system with the origin [phi,lambda]'

    phi = ned_lla(1);
    lambda = ned_lla(2);

    % transformation  matrix
    T = [-sin(phi)*cos(lambda) -sin(phi)*sin(lambda)  cos(phi)
         -sin(lambda)           cos(lambda)           0
          cos(phi)*cos(lambda)   cos(phi)*sin(lambda)  sin(phi)];

     x_ned = T*(x_ecef-lla2ecef([phi, lambda, 0]')); % convert to NED
     x_ned(3) = -x_ned(3);
end
